simulink library "Mylibrary"  (Simulink 8.3)
settings: Solver=ode45  StartTime=0.0  StopTime=10.0  RelTol=1e-3
undefined symbols (not defined in the file or in its folder): Delay, epsilon, L, Mode, R, T_Trigger, tau_bar, Ts, Ts1, vd, Vehicle_Index, vp, x0, y0
undefined symbols (not defined in the file): d1, m1, psi20, Vx, Vy, x20, y20
libraries: Mylibrary x3
(part 3 of 3)

== matlab function CPF Lapier Miguel Hung  ==
  settings: updateMethod=DISCRETE  sampleTime=0.2
  data: t input double; Re_Data1 input double; Re_Data2 input double; Com_Sig input double; tau_bar parameter double; DataToTran output double; p input double size=2; r input double; yaw input double size=1; u input double size=1; gamma_c output double size=1; vcxy_hat output double; yaw_ref output double; r_ref output double; precise output double; u_ref output double; pd output double; L parameter double; R parameter double; d parameter double; m parameter double; vp parameter double; gamma_dot output double
function [DataToTran,gamma_c,vcxy_hat,yaw_ref,r_ref,precise,u_ref,pd,gamma_dot] = fcn(t,Re_Data1,Re_Data2,Com_Sig,tau_bar,p,r,yaw,u,L, R, d, m, vp)
%% declare variables
    persistent  gamma gamma_c_M 
    persistent vcx vcy
    if isempty (gamma)
         gamma=0; gamma_c_M=0;                                 % we can start any value of gamma here
         vcx=0;vcy=0;
    end
%% In first 2 seconds, do nothing, just wait for estimation of GPS, sensors    
    if t<2
        DataToTran=[0;0];
        gamma_c=0;
        vcxy_hat=[0;0];
        yaw_ref=0;
        r_ref=0;
        precise=0;
        u_ref=0;    
        pd=[0;0];
        gamma_dot=0;
    else
%% After two senconds, do the job    
%-------------------
    Ts=0.2; 
% Update the path and coordination state gamma_c
    [gamma_c,vd_bar,path_point] = path(gamma,L, R, d, m, vp);
    pd=[path_point(1);path_point(2)]; 
    theta_c=path_point(3)*180/pi;
    c_c=path_point(5);
    g_c=path_point(6);
    s_dot=path_point(7);
    s_ddot=path_point(8);
% Calculate correction speed from coordination law  
    v_comp=norm([vp*cosd(yaw)+vcx vp*sind(yaw)+vcy]);
    [vd_t,DataToTran] = Coordination(t,gamma_c,gamma_c_M,Re_Data1,Re_Data2,Com_Sig,tau_bar,vp,v_comp,vd_bar);
% Implement Path Following Controller
    vd=vd_bar+0*vd_t;
    [gamma_next,vcxy_hat,yaw_ref,r_ref,precise,u_ref,pd,gamma_dot] = PF(vd,p,r,yaw,u,theta_c,c_c,g_c,pd,s_dot,s_ddot,t);
% Update gamma_c_M
    gamma_c_M=gamma_c;
    gamma=gamma_next;
    vcx=vcxy_hat(1);
    vcy=vcxy_hat(2);
%---------------------
    end
end

function [gamma_next,vcxy_hat,yaw_ref,r_ref,precise,u_ref,pd,gamma_dot] = PF(vd,p,r,yaw,u,theta_c,c_c,g_c,pd,s_dot,s_ddot,t)

%% Declare and initialize global variales                                   These variables will be kept in memory during execuation
    Ts=0.2;         
    persistent vr_hat_old   vr_hat    % sampling time
    persistent p_hat_old    p_hat   Vcxy_hat_old Vcxy_hat 
    persistent gamma 
    if isempty(p_hat)
        vr_hat_old=0;            vr_hat=0; 
        p_hat=p;                 p_hat_old=p;    Vcxy_hat_old=[0;0];  Vcxy_hat=[0;0];
        gamma=0;  
    end    
%% Vehicle Prameters
    mass = 17.0;
    X_dot_u = -20;
    Y_dot_v = -30;                                                              %-1.3175;
    Y_v = -50;
    Y_vv = -0.01;                                                               %-101.2776;
    % masses
    m_u = mass - X_dot_u;
    m_v = mass - Y_dot_v;
    N_r = -4.14; %-0.1
    N_rr = -6.23; %-21
%% error between vehicle and rabbit
   R1=[cosd(theta_c)       sind(theta_c);     % From {I} to {F}
      -sind(theta_c)       cosd(theta_c)]; 
   e=p-pd;
   e_f=R1*e;
   s1=e_f(1);
   y1=e_f(2);      
%% Estimate vr
    d_v = -Y_v - Y_vv*abs(vr_hat);
    vr_hat_dot=-m_u*u*r/m_v-d_v*vr_hat/m_v;
    vr_hat=vr_hat_old+Ts*vr_hat_dot;
    vr_hat_old=vr_hat; 
%% Estimate current 
% Estimate current in Inertial frame
    R2=[cosd(yaw)        -sind(yaw);     % From {B} to {I}
        sind(yaw)         cosd(yaw)]; 
    p_t=p-p_hat;
    Vr=[u;0*vr_hat];
    Kp=10*[1 0;
           0 1];
    Kc=10*[1 0;
          0 1];
    p_hat_dot=R2*Vr+Vcxy_hat+Kp*p_t;
    p_hat=p_hat_old+Ts*p_hat_dot;
    p_hat_old=p_hat;
    Vcxy_hat_dot=Kc*p_t;
    Vcxy_hat=Vcxy_hat_old+Ts*Vcxy_hat_dot;
    Vcxy_hat_old=Vcxy_hat;
    vcxy_hat=Vcxy_hat;
% Transform the estimated current to Frenet frame
    Vc_hat_f=R1*Vcxy_hat;                      
    Vc_par=Vc_hat_f(1);
    Vc_per=Vc_hat_f(2);
%% Outerloop Controller
   s=8;
   if t<=20;
       m=0.05*t;
   else
       m=1;
   end
   a=y1/s+m*Vc_per/u;
%    a=y1/s;                                             % No current                          
   a= min(max(a, -1), 1);
   theta=-asind(a);
% Yaw reference
   yaw_ref=theta_c+theta;
%    yaw_ref=60;
% Yaw rate reference
    r_ref=-c_c*s_dot*180/pi;
%     r_ref=0;
% speed reference

%      R3=[cosd(yaw)         sind(yaw);     % From {B} to {I}
%          -sind(yaw)         cosd(yaw)]; 
     u_ref=vd;
%% Gamma Controller
   k1=1;
   gamma_dot=u*cosd(yaw-theta_c)+k1*s1+Vc_par;
%       gamma_dot=vd*cosd(yaw-theta_c)+k1*s1;
%    if gamma_dot<=0
%        gamma_dot=0;
%    end
   gamma_next=gamma+Ts*gamma_dot;
   gamma=gamma_next;
% Precicise 
    r_rad=r*pi/180;
    precise=-g_c*s_dot^2-c_c*s_ddot - N_r*r_rad - N_rr*r_rad*abs(r_rad);
%     precise=0;
end
%%-------------------------------------------------------------------------------------------------------------
%%-------------------------------------------------------------------------------------------------------------
function [vd_t,DataToTran,e_int] = Coordination(t,gamma_c,gamma_c_M,Re_Data1,Re_Data2,Com_Sig,tau_bar,vp,v_comp,vd_bar)

%% Declare variables
    persistent gamma_cn1 gamma_cn2 gamma_c0 tc1 tc2 tcn11 tcn12 tcn21 tcn22 tem_c tem_cn1 tem_cn2 reset_c reset_cn1 reset_cn2 e_int_t;   
    if isempty(gamma_cn1)
        gamma_cn1=0;gamma_cn2=0;
        gamma_c0=0;
        tcn11=t;tcn12=t;
        tcn21=t;tcn22=t;
        tc1=t;tc2=t;
        tem_c=t;
        tem_cn1=t;tem_cn2=t;
        reset_c=false;
        reset_cn1=false;
        reset_cn2=false;
        e_int_t=0;
    end
%% Reset estimator for gamma_c of first neighbor;
    if (Re_Data1(1)~=0)                                  % If recived new data, reset estimator that the current vehicle thinks about the neighbor vehicle
        tcn11=Re_Data1(1); 
        tem_cn1=Re_Data1(2);
        reset_cn1=true;
    end   
    if (t-tcn11>tau_bar)&&reset_cn1
        gamma_cn1=tem_cn1+vp*tau_bar;
%         gamma_cn1=tem_cn1+vd_bar*tau_bar;
        reset_cn1=false;
        tcn12=t;
    end
%% Reset estimator for gamma_c of second neighbor;
    if (Re_Data2(1)~=0)                                  % If recived new data, reset estimator that the current vehicle thinks about the neighbor vehicle
        tcn21=Re_Data2(1); 
        tem_cn2=Re_Data2(2);
        reset_cn2=true;
    end   
    if (t-tcn21>tau_bar)&&reset_cn2
        gamma_cn2=tem_cn2+vp*tau_bar;
%         gamma_cn2=tem_cn2+vd_bar*tau_bar;

        reset_cn2=false;
        tcn22=t;
    end
%% Reset estimator for gamma_c of current vehicle   % When it sends its coordinate state to neighbor, it needs to update its estimator too to synchoronize with the neighbor
    if (Com_Sig~=0)
        tc1=t;
        tem_c=gamma_c;
        reset_c=true;
    end
    if (t-tc1>tau_bar)&& reset_c
        gamma_c0=tem_c+vp*tau_bar;
%                 gamma_c0=tem_c+vd_bar*tau_bar;

        reset_c=false;
        tc2=t;
    end
%% Run estimators of gamma
       gamma_c_hat=gamma_c0+vp*(t-tc2);
       gamma_c_n1_hat=gamma_cn1+vp*(t-tcn12);
       gamma_c_n2_hat=gamma_cn2+vp*(t-tcn22);
%      gamma_c_hat=gamma_c0+vd_bar*(t-tc2);
%      gamma_c_n1_hat=gamma_cn1+vd_bar*(t-tcn12);
%      gamma_c_n2_hat=gamma_cn2+vd_bar*(t-tcn22);
%% Accumulate error for integration term
    Ts=0.2;
    if (Re_Data1(2)~=0)                                                    % accumulate error when recieve new data from neigbor
       e=gamma_c_M-Re_Data1(2);
       e_int_t=e_int_t+.5*Ts*e;
    end
    if (Re_Data2(2)~=0) 
       e=gamma_c_M-Re_Data2(2);
       e_int_t=e_int_t+.5*Ts*e;
    end
%% Compute correction term 
    kg=.1;
    ki=.00;
    e1=(gamma_c_M-0.5*(gamma_c_n1_hat+gamma_c_n2_hat));
%     e1=(gamma_c_M-0.5*(Re_Data1(2)+Re_Data2(2)));
    vd_t=-kg*e1-ki*e_int_t;
    vd_t_max=vp;
    vd_t_min=-vp;
    if  vd_t<vd_t_min;
        vd_t=vd_t_min;
    elseif vd_t>=vd_t_max
        vd_t=vd_t_max;
    end
    e_int=e_int_t;
%% Prepare Data for transmition block
    gamma_e=gamma_c-gamma_c_hat;
    DataToTran=[gamma_c;gamma_e];
end
%%-------------------------------------------------------------------------------------------------------------
%%-------------------------------------------------------------------------------------------------------------
function [gamma_c,vd_bar,path_point] = path(gamma,L, R, d, m, vp) 
%% Path parameters
Ts=0.2;
s1=L-m;
s2=s1+pi*(R-d);
s3=s2+L;
s4=s3+pi*(R+d);
s5=s4+m;
ratio1=(R-d)/R;
ratio2=(R+d)/R;
% ratio1=1;
% ratio2=1;
if gamma<s5;
    cycle=0;
else
    cycle=1;
end
s=gamma-s5*cycle;
%% Declaration variable to calculate s_dot, s_ddot
persistent c_c_old gamma_old s_dot_old
if isempty(c_c_old)
    c_c_old=0;
    gamma_old=0;
    s_dot_old=0;
end
%% Update path information depending upon on gamma (or s)
if s<s1                                    % first segment of straight line;
    vd_bar=vp;
    xd=0+d;
    yd=s+R+m;
    theta_c=pi/2;
    gamma_c=s+s5*cycle;                    % the segment is parallel with x
    c_c=0;
elseif (s>=s1) && (s<=s2)                  % second segment, a circumference 
    vd_bar=ratio1*vp;
    theta_c=pi/2-(s-s1)/((R-d));
    xd=d+(R-d)*(1-sin(theta_c));
    yd=L+R+(R-d)*cos(theta_c);   
    gamma_c=s1+(s-s1)*R/(R-d)+s5*cycle; 
    c_c=1/(R-d);
elseif (s>s2) && (s<=s3)                   % third segment, a straight line 
    vd_bar=vp;
    yd=s3-s+R;  
    theta_c=-pi/2;
    xd=d+2*(R-d);
    gamma_c=s+d*pi+s5*cycle;
    c_c=0;
elseif (s>s3) && (s<=s4)   
    vd_bar=ratio2*vp;
    theta_c=-pi/2+(s-s3)/(R+d);
    xd=d+2*(R-d)+(R+d)*(1+sin(theta_c));
    yd=R-(R+d)*cos(theta_c);
    gamma_c=s3+d*pi+(s-s3)*R/(R+d)+s5*cycle;   
    c_c=-1/(R+d);
else
    vd_bar=vp;
    yd=(s-s4)+R;
    xd=d+4*R;
    theta_c=pi;
    gamma_c=s+s5*cycle;
    c_c=0;
end
%% Caculate s_dot,sddot,g_c

c_c_dot=c_c-c_c_old;
s_dot=(gamma-gamma_old)/Ts;
s_ddot=(s_dot-s_dot_old)/Ts;
                                                        % g_c=c_c_dot/s_dot;
if s_dot==0
    g_c=0;
else
    g_c=c_c_dot/s_dot; 
end   
%%      
c_c_old=c_c;
gamma_old=gamma;
s_dot_old=s_dot;
path_point=[cycle*4*R+xd,yd,theta_c,gamma,c_c,g_c,s_dot,s_ddot];
end

== matlab function CPF Lapier Miguel Hung Current ==
  settings: updateMethod=DISCRETE  sampleTime=0.2
  data: t input double; Re_Data1 input double; Re_Data2 input double; Com_Sig input double; tau_bar parameter double; DataToTran output double; p input double size=2; r input double; yaw input double size=1; u input double size=1; gamma_c output double size=1; vcxy_hat output double; yaw_ref output double; r_ref output double; precise output double; u_ref output double; pd output double; L parameter double; R parameter double; d parameter double; m parameter double; vp parameter double; gamma_dot output double
function [DataToTran,gamma_c,vcxy_hat,yaw_ref,r_ref,precise,u_ref,pd,gamma_dot] = fcn(t,Re_Data1,Re_Data2,Com_Sig,tau_bar,p,r,yaw,u,L, R, d, m, vp)
%% declare variables
    persistent  gamma gamma_c_M 
    persistent vcx vcy
    if isempty (gamma)
         gamma=0; gamma_c_M=0;                                 % we can start any value of gamma here
         vcx=0;vcy=0;
    end
%% In first 2 seconds, do nothing, just wait for estimation of GPS, sensors    
    if t<2
        DataToTran=[0;0];
        gamma_c=0;
        vcxy_hat=[0;0];
        yaw_ref=0;
        r_ref=0;
        precise=0;
        u_ref=0;    
        pd=[0;0];
        gamma_dot=0;
    else
%% After two senconds, do the job    
%-------------------
    Ts=0.2; 
% Update the path and coordination state gamma_c
    [gamma_c,vd_bar,path_point] = path(gamma,L, R, d, m, vp);
    pd=[path_point(1);path_point(2)]; 
    theta_c=path_point(3)*180/pi;
    c_c=path_point(5);
    g_c=path_point(6);
    s_dot=path_point(7);
    s_ddot=path_point(8);
% Calculate correction speed from coordination law  
    v_comp=norm([vp*cosd(yaw)+vcx vp*sind(yaw)+vcy]);
    [vd_t,DataToTran] = Coordination(t,gamma_c,gamma_c_M,Re_Data1,Re_Data2,Com_Sig,tau_bar,vp,v_comp,vd_bar);
% Implement Path Following Controller
    vd=vd_bar+0*vd_t;
    [gamma_next,vcxy_hat,yaw_ref,r_ref,precise,u_ref,pd,gamma_dot] = PF(vd,p,r,yaw,u,theta_c,c_c,g_c,pd,s_dot,s_ddot,t);
% Update gamma_c_M
    gamma_c_M=gamma_c;
    gamma=gamma_next;
    vcx=vcxy_hat(1);
    vcy=vcxy_hat(2);
%---------------------
    end
end

function [gamma_next,vcxy_hat,yaw_ref,r_ref,precise,u_ref,pd,gamma_dot] = PF(vd,p,r,yaw,u,theta_c,c_c,g_c,pd,s_dot,s_ddot,t)

%% Declare and initialize global variales                                   These variables will be kept in memory during execuation
    Ts=0.2;         
    persistent vr_hat_old   vr_hat    % sampling time
    persistent p_hat_old    p_hat   Vcxy_hat_old Vcxy_hat 
    persistent gamma 
    if isempty(p_hat)
        vr_hat_old=0;            vr_hat=0; 
        p_hat=p;                 p_hat_old=p;    Vcxy_hat_old=[0;0];  Vcxy_hat=[0;0];
        gamma=0;  
    end    
%% Vehicle Prameters
    mass = 17.0;
    X_dot_u = -20;
    Y_dot_v = -30;                                                              %-1.3175;
    Y_v = -50;
    Y_vv = -0.01;                                                               %-101.2776;
    % masses
    m_u = mass - X_dot_u;
    m_v = mass - Y_dot_v;
    N_r = -4.14; %-0.1
    N_rr = -6.23; %-21
%% error between vehicle and rabbit
   R1=[cosd(theta_c)       sind(theta_c);     % From {I} to {F}
      -sind(theta_c)       cosd(theta_c)]; 
   e=p-pd;
   e_f=R1*e;
   s1=e_f(1);
   y1=e_f(2);      
%% Estimate vr
    d_v = -Y_v - Y_vv*abs(vr_hat);
    vr_hat_dot=-m_u*u*r/m_v-d_v*vr_hat/m_v;
    vr_hat=vr_hat_old+Ts*vr_hat_dot;
    vr_hat_old=vr_hat; 
%% Estimate current 
% Estimate current in Inertial frame
    R2=[cosd(yaw)        -sind(yaw);     % From {B} to {I}
        sind(yaw)         cosd(yaw)]; 
    p_t=p-p_hat;
    Vr=[u;0*vr_hat];
    Kp=5*[1 0;
           0 1];
    Kc=5*[1 0;
          0 1];
    p_hat_dot=R2*Vr+Vcxy_hat+Kp*p_t;
    p_hat=p_hat_old+Ts*p_hat_dot;
    p_hat_old=p_hat;
    Vcxy_hat_dot=Kc*p_t;
    Vcxy_hat=Vcxy_hat_old+Ts*Vcxy_hat_dot;
    Vcxy_hat_old=Vcxy_hat;
    vcxy_hat=Vcxy_hat;

%% Outerloop Controller
   s=6;
   if t<=50;
       m=0.02*t;
   else
       m=1;
   end
   a=m*y1/s;
%    a=y1/s;                                             % No current                          
   a= min(max(a, -1), 1);
   % compute alpha
   phi_e=atan2d((u*sind(yaw)+Vcxy_hat(2)),(u*cosd(yaw)+Vcxy_hat(1)));
   alpha=phi_e-yaw; 
   beta_d=-asind(a);
   phi_e_ref=theta_c+beta_d;
% Yaw reference
   yaw_ref=phi_e_ref-alpha;
%    yaw_ref=60;
% Yaw rate reference
    r_ref=-c_c*s_dot*180/pi;
%     r_ref=0;
% speed reference

%      R3=[cosd(yaw)         sind(yaw);     % From {B} to {I}
%          -sind(yaw)         cosd(yaw)]; 
     u_ref=vd;
%% Gamma Controller
   k1=1;
   beta=phi_e-theta_c;
   gamma_dot=u_ref*cosd(beta)+k1*s1;
%       gamma_dot=vd*cosd(yaw-theta_c)+k1*s1;
%    if gamma_dot<=0
%        gamma_dot=0;
%    end
   gamma_next=gamma+Ts*gamma_dot;
   gamma=gamma_next;
% Precicise 
    r_rad=r*pi/180;
    precise=-g_c*s_dot^2-c_c*s_ddot - N_r*r_rad - N_rr*r_rad*abs(r_rad);
%     precise=0;
end
%%-------------------------------------------------------------------------------------------------------------
%%-------------------------------------------------------------------------------------------------------------
function [vd_t,DataToTran,e_int] = Coordination(t,gamma_c,gamma_c_M,Re_Data1,Re_Data2,Com_Sig,tau_bar,vp,v_comp,vd_bar)

%% Declare variables
    persistent gamma_cn1 gamma_cn2 gamma_c0 tc1 tc2 tcn11 tcn12 tcn21 tcn22 tem_c tem_cn1 tem_cn2 reset_c reset_cn1 reset_cn2 e_int_t;   
    if isempty(gamma_cn1)
        gamma_cn1=0;gamma_cn2=0;
        gamma_c0=0;
        tcn11=t;tcn12=t;
        tcn21=t;tcn22=t;
        tc1=t;tc2=t;
        tem_c=t;
        tem_cn1=t;tem_cn2=t;
        reset_c=false;
        reset_cn1=false;
        reset_cn2=false;
        e_int_t=0;
    end
%% Reset estimator for gamma_c of first neighbor;
    if (Re_Data1(1)~=0)                                  % If recived new data, reset estimator that the current vehicle thinks about the neighbor vehicle
        tcn11=Re_Data1(1); 
        tem_cn1=Re_Data1(2);
        reset_cn1=true;
    end   
    if (t-tcn11>tau_bar)&&reset_cn1
        gamma_cn1=tem_cn1+vp*tau_bar;
%         gamma_cn1=tem_cn1+vd_bar*tau_bar;
        reset_cn1=false;
        tcn12=t;
    end
%% Reset estimator for gamma_c of second neighbor;
    if (Re_Data2(1)~=0)                                  % If recived new data, reset estimator that the current vehicle thinks about the neighbor vehicle
        tcn21=Re_Data2(1); 
        tem_cn2=Re_Data2(2);
        reset_cn2=true;
    end   
    if (t-tcn21>tau_bar)&&reset_cn2
        gamma_cn2=tem_cn2+vp*tau_bar;
%         gamma_cn2=tem_cn2+vd_bar*tau_bar;

        reset_cn2=false;
        tcn22=t;
    end
%% Reset estimator for gamma_c of current vehicle   % When it sends its coordinate state to neighbor, it needs to update its estimator too to synchoronize with the neighbor
    if (Com_Sig~=0)
        tc1=t;
        tem_c=gamma_c;
        reset_c=true;
    end
    if (t-tc1>tau_bar)&& reset_c
        gamma_c0=tem_c+vp*tau_bar;
%                 gamma_c0=tem_c+vd_bar*tau_bar;

        reset_c=false;
        tc2=t;
    end
%% Run estimators of gamma
       gamma_c_hat=gamma_c0+vp*(t-tc2);
       gamma_c_n1_hat=gamma_cn1+vp*(t-tcn12);
       gamma_c_n2_hat=gamma_cn2+vp*(t-tcn22);
%      gamma_c_hat=gamma_c0+vd_bar*(t-tc2);
%      gamma_c_n1_hat=gamma_cn1+vd_bar*(t-tcn12);
%      gamma_c_n2_hat=gamma_cn2+vd_bar*(t-tcn22);
%% Accumulate error for integration term
    Ts=0.2;
    if (Re_Data1(2)~=0)                                                    % accumulate error when recieve new data from neigbor
       e=gamma_c_M-Re_Data1(2);
       e_int_t=e_int_t+.5*Ts*e;
    end
    if (Re_Data2(2)~=0) 
       e=gamma_c_M-Re_Data2(2);
       e_int_t=e_int_t+.5*Ts*e;
    end
%% Compute correction term 
    kg=.2;
    ki=.00;
    e1=(gamma_c_M-0.5*(gamma_c_n1_hat+gamma_c_n2_hat));
%     e1=(gamma_c_M-0.5*(Re_Data1(2)+Re_Data2(2)));
    vd_t=-kg*e1-ki*e_int_t;
    vd_t_max=vp;
    vd_t_min=-vp;
    if  vd_t<vd_t_min;
        vd_t=vd_t_min;
    elseif vd_t>=vd_t_max
        vd_t=vd_t_max;
    end
    e_int=e_int_t;
%% Prepare Data for transmition block
    gamma_e=gamma_c-gamma_c_hat;
    DataToTran=[gamma_c;gamma_e];
end
%%-------------------------------------------------------------------------------------------------------------
%%-------------------------------------------------------------------------------------------------------------
function [gamma_c,vd_bar,path_point] = path(gamma,L, R, d, m, vp) 
%% Path parameters
Ts=0.2;
s1=L-m;
s2=s1+pi*(R-d);
s3=s2+L;
s4=s3+pi*(R+d);
s5=s4+m;
ratio1=(R-d)/R;
ratio2=(R+d)/R;
% ratio1=1;
% ratio2=1;
if gamma<s5;
    cycle=0;
else
    cycle=1;
end
s=gamma-s5*cycle;
%% Declaration variable to calculate s_dot, s_ddot
persistent c_c_old gamma_old s_dot_old
if isempty(c_c_old)
    c_c_old=0;
    gamma_old=0;
    s_dot_old=0;
end
%% Update path information depending upon on gamma (or s)
if s<s1                                    % first segment of straight line;
    vd_bar=vp;
    xd=0+d;
    yd=s+R+m;
    theta_c=pi/2;
    gamma_c=s+s5*cycle;                    % the segment is parallel with x
    c_c=0;
elseif (s>=s1) && (s<=s2)                  % second segment, a circumference 
    vd_bar=ratio1*vp;
    theta_c=pi/2-(s-s1)/((R-d));
    xd=d+(R-d)*(1-sin(theta_c));
    yd=L+R+(R-d)*cos(theta_c);   
    gamma_c=s1+(s-s1)*R/(R-d)+s5*cycle; 
    c_c=1/(R-d);
elseif (s>s2) && (s<=s3)                   % third segment, a straight line 
    vd_bar=vp;
    yd=s3-s+R;  
    theta_c=-pi/2;
    xd=d+2*(R-d);
    gamma_c=s+d*pi+s5*cycle;
    c_c=0;
elseif (s>s3) && (s<=s4)   
    vd_bar=ratio2*vp;
    theta_c=-pi/2+(s-s3)/(R+d);
    xd=d+2*(R-d)+(R+d)*(1+sin(theta_c));
    yd=R-(R+d)*cos(theta_c);
    gamma_c=s3+d*pi+(s-s3)*R/(R+d)+s5*cycle;   
    c_c=-1/(R+d);
else
    vd_bar=vp;
    yd=(s-s4)+R;
    xd=d+4*R;
    theta_c=pi;
    gamma_c=s+s5*cycle;
    c_c=0;
end
%% Caculate s_dot,sddot,g_c

c_c_dot=c_c-c_c_old;
s_dot=(gamma-gamma_old)/Ts;
s_ddot=(s_dot-s_dot_old)/Ts;
                                                        % g_c=c_c_dot/s_dot;
if s_dot==0
    g_c=0;
else
    g_c=c_c_dot/s_dot; 
end   
%%      
c_c_old=c_c;
gamma_old=gamma;
s_dot_old=s_dot;
path_point=[cycle*4*R+xd,yd,theta_c,gamma,c_c,g_c,s_dot,s_ddot];
end

== matlab function Kinematic Model/Kinematic Model ==
  data: u input double; x_dot output double; yaw input double; y_dot output double
function [x_dot, y_dot] = fcn(u, yaw)
x_dot=u*cos(yaw);
y_dot=u*sin(yaw);

== matlab function Simplified CPF Controller Latest version  ==
  settings: updateMethod=DISCRETE  sampleTime=0.2
  data: t input double size=1; Re_Data1 input double size=2; Re_Data2 input double size=2; u input double size=1; r input double size=1; yaw input double size=1; p input double size=2; L parameter double size=1; R parameter double size=1; d parameter double size=1; m parameter double size=1; u_d output double size=1; r_d output double size=1; Com_Mode output double size=1; Diff_Mode output double size=1; DatatoTran output double size=2; vd_t output double size=1; vp parameter double size=1; pd output double size=2; Mode parameter double; T_Trigger parameter double; epsilon parameter double; tau_bar parameter double
%% CPF is main function for Event/Time Trigger Coordinated Pathfollowing
function [u_d,r_d,Com_Mode,Diff_Mode,DatatoTran,vd_t,pd] = CPF(t,Re_Data1,Re_Data2,u,r,yaw,p,L, R, d,m,vp, Mode,T_Trigger,epsilon,tau_bar)
%% Declare variables
persistent  gamma gamma_c_M 
persistent  Com_Sig
if isempty (gamma)
         gamma=0; gamma_c_M=0;                                              % Noted that we can start any value of gamma here
         Com_Sig=0;   
end
if t<5                                                                      % Wait for update GPS... I am not sure, must be confirmed by experts            
    Com_Mode=0;Diff_Mode=0;
    DatatoTran=[0;0];  
    u_d=0;
    r_d=0;
    vd_t=0;
    pd=[0;0];
else
% Update the path and coordination state gamma_c
    [gamma_c,pd,pd_gamma,vd_bar,cur] = path(gamma,vp,L,R,d,m);
    
%% Calculate correction speed from coordination law
    Ts=0.2; 
    % Step 1: Run internal estimator to estimate neigbor's coordination state
     [gamma_c_hat,gamma_c_n1_hat,gamma_c_n2_hat] = Int_Est(t,gamma_c,Re_Data1,Re_Data2,vp,Com_Sig,tau_bar);   
    % Step 2: Call Coordination rule
      vd_t = Coordination(gamma_c,gamma_c_M,Re_Data1,Re_Data2,gamma_c_n1_hat,gamma_c_n2_hat,vp);

%% Transmit data (time and coordinated state (normalized) to neighbor)
  [DatatoTran,Com_Sig] = Trans(t,gamma_c,gamma_c_hat, Mode,T_Trigger,epsilon,tau_bar);
%% Implement Path Following Controller
%     vd_t=0;
  [gamma_next,u_d,r_d,Com_Mode,Diff_Mode] = PF(t,pd,pd_gamma,vd_bar,vd_t,u,r,yaw,p,Ts,cur);
    
%% Update
    gamma_c_M=gamma_c;
    gamma=gamma_next;
end
end
    %% PF function is for Path Flollowing Controller                                  
    function [gamma_next,u_d,r_d,Com_Mode,Diff_Mode] = PF(t,pd,pd_gamma,vd_bar,vd_t,u,r,yaw,p,Ts,cur)

    %% Declare and initialize global variales                                   These variables will be kept in memory during execuation
        persistent p_hat_old    p_hat   Vcxy_hat_old Vcxy_hat 
        persistent gamma_dot_old gamma_dot gamma_old
        persistent ud_t
        persistent eu_old Com_Mode_old
        persistent er_old Diff_Mode_old
        persistent vd_old vd_new
        if isempty(p_hat_old)
            p_hat=p;                p_hat_old=p;    Vcxy_hat_old=[0;0];  Vcxy_hat=[0;0];
            gamma_dot_old=0;        gamma_dot=0;    gamma_old=0;
            eu_old=0; Com_Mode_old=0;
            er_old=0; Diff_Mode_old=0;
            vd_old=0; vd_new=0;
            lock=0;
        end

    %% Calculate rotation matrix from body frame to inertial frame

        R=[cosd(yaw)   -sind(yaw);
           sind(yaw)    cosd(yaw)]; 

    %% Estimate current 
    % Estimate current in Inertial frame
        p_t=p-p_hat;
        Vr=[u;0];
        Kp=10*[1 0;
               0 1];
        Kc=10*[1 0;
              0 1];
        p_hat_dot=R*Vr+Vcxy_hat+Kp*p_t;
        p_hat=p_hat_old+Ts*p_hat_dot;
        p_hat_old=p_hat;
        Vcxy_hat_dot=Kc*p_t;
        Vcxy_hat=Vcxy_hat_old+Ts*Vcxy_hat_dot;
        Vcxy_hat_old=Vcxy_hat;
    % Transform the estimated current to Body frame
        Vc_hat=R'*Vcxy_hat;

    %% Outerloop Controller
        vd=vd_bar+vd_t;
        e_out=R'*(p-pd);
        delta=-0.2;
        Delta_inv= 1*[1    0;
                      0 -1/delta];     

        if t<30
            kx=0.01*t;
            ky=0.006*t;
            m=.0017*t;
        else
            kx=0.3;
            ky=0.2;
            m=0.05;
        end
         
          Kk=[kx+cur 0;
            0  ky+cur];
          ud_t=Delta_inv*(-Kk*tanh(e_out-[delta;0])-Vc_hat+R'*pd_gamma*vd);  
          n=1;
         
          ud=[n 0; 0 m+cur]*ud_t;
          u_d=ud(1);
          r_d=ud(2)*180/(pi); 
    %% Inner Loop Controller
        eu=u_d-u;
        er=r_d-r;
        % Speed controller
        Kp_u=30;
        KI_u=10;
        KD_u=0;
        Com_Mode=Kp_u*eu+(Ts*KI_u-Kp_u)*eu_old+Com_Mode_old;
        Com_Mode_old=Com_Mode;
        eu_old=eu;
        % Yaw rate controller
        Kp_r=10;
        KI_r=2;
        KD_r=0;
        Diff_Mode=Kp_r*er+(Ts*KI_r-Kp_r)*er_old+Diff_Mode_old;
        Diff_Mode_old=Diff_Mode;
        er_old=er;

    %% Gamma Controller
        kz=1;
        vd_dot=(vd_new-vd_old)/Ts;   
        vd_old=vd_new;
        gamma_ddot=-kz*(gamma_dot-vd_bar)+vd_dot+2*(e_out-[delta;0])'*R'*pd_gamma + 1*kz*vd_t; 
        gamma_dot=gamma_dot_old+Ts*gamma_ddot;
        gamma_next=gamma_old+Ts*gamma_dot;
        gamma_dot_old=gamma_dot;
        gamma_old=gamma_next;
    end                 
    %% Coordinaiton function is for Time/Event Trigger Cordination Law
    function vd_t = Coordination(gamma_c,gamma_c_M,Re_Data1,Re_Data2,gamma_c_n1_hat,gamma_c_n2_hat,vp)
       persistent e_int;
       if isempty (e_int)
           e_int=0;
       end
    %% Accumulate error for integration term
        Ts=0.2;
        if (Re_Data1(2)~=0)                                                    % accumulate error when recieve new data from neigbor
           e=gamma_c_M-Re_Data1(2);
           e_int=e_int+.5*Ts*e;
        end
        if (Re_Data2(2)~=0) 
           e=gamma_c_M-Re_Data2(2);
           e_int=e_int+.5*Ts*e;
        end
    %% Compute correction term 
        kg=.1;
        ki=.000;
        e1=(gamma_c-0.5*(gamma_c_n1_hat+gamma_c_n2_hat));
    %     e1=(gamma_c_M-0.5*(Re_Data1(2)+Re_Data2(2)));
        vd_t=-kg*e1-ki*e_int;
    %   Put saturation to avoid the vehicle return back.    
        vd_t_max=vp;
        vd_t_min=-vp;
        if  vd_t<vd_t_min;
            vd_t=vd_t_min;
        elseif vd_t>=vd_t_max
            vd_t=vd_t_max;
        end
    end
    %% Internal Estimator
    function [gamma_c_hat,gamma_c_n1_hat,gamma_c_n2_hat] = Int_Est(t,gamma_c,Re_Data1,Re_Data2,vp,Com_Sig,tau_bar)                                                       % No delay
    %% Declare variables
        persistent gamma_cn1 gamma_cn2 gamma_c0 tc2 tcn12 tcn22 tem_c tem_cn1 tem_cn2   
        if isempty(gamma_cn1)
            gamma_cn1=0;gamma_cn2=0;
            gamma_c0=0;
            tcn12=t;
            tcn22=t;
            tc2=t;
            tem_c=t;
            tem_cn1=t;tem_cn2=t;
        end
    %% Reset estimator for gamma_c of first neighbor;
        if (Re_Data1(1)~=0)                                  % If recived new data, reset estimator that the current vehicle thinks about the neighbor vehicle
            tem_cn1=Re_Data1(2);
            gamma_cn1=tem_cn1+vp*tau_bar;                    % Compensate tau_bar is the delay time for transmition 
            tcn12=t;
        end
    %% Reset estimator for gamma_c of second neighbor;
        if (Re_Data2(1)~=0)                                  % If recived new data, reset estimator that the current vehicle thinks about the neighbor vehicle
            tem_cn2=Re_Data2(2);
            gamma_cn2=tem_cn2+vp*tau_bar;
            tcn22=t;
        end
    %% Reset estimator for gamma_c of current vehicle        % When the vehicle sends its coordinate state to neighbors, it needs to update its estimator too to synchoronize with its neighbors
        if (Com_Sig~=0)
            tem_c=gamma_c;
            gamma_c0=tem_c;
            tc2=t;
        end
    %% Run estimators of gamma
        gamma_c_hat=gamma_c0+vp*(t-tc2);
        gamma_c_n1_hat=gamma_cn1+vp*(t-tcn12);
        gamma_c_n2_hat=gamma_cn2+vp*(t-tcn22); 
end
    %% Path function is path generator (Lawn mower)
    function [gamma_c,pd,pd_gamma,vd_bar,cur] = path(gamma,vp,L,R,d,m) 
    s1=L-m;
    s2=s1+pi*(R-d);
    s3=s2+L;
    s4=s3+pi*(R+d);
    s5=s4+m;
    ratio1=(R-d)/R;
    ratio2=(R+d)/R;
%     ratio1=1;
%     ratio2=1;

    if gamma<s5;
        cycle=0;
    else
        cycle=1;
    end
    s=gamma-s5*cycle;
    c1=1.2/(R-d);
    c2=1/(R+d);
    k=.5;
    cur=c1/(1+exp(-k*(s-s1)))-c1/(1+exp(-k*(s-s2)))+c2/(1+exp(-k*(s-s3)))-c2/(1+exp(-k*(s-s4)));
    if s<s1                                    % first segment of straight line;
        vd_bar=vp;
        xd=s+R+m;
        yd=0+d;
        pd_gamma=[1;0];      
        gamma_c=s+s5*cycle;                                  % the segment is parallel with x
    elseif (s>=s1) && (s<=s2)                  % second segment, a circumference 
        vd_bar=ratio1*vp;
        psi_T=(s-s1)/(R-d);
        xd=L+R+(R-d)*sin(psi_T);   
        yd=d+(R-d)*(1-cos(psi_T));
        pd_gamma=[cos(psi_T);sin(psi_T)];
        gamma_c=s1+(s-s1)*R/(R-d)+s5*cycle; 
    elseif (s>s2) && (s<=s3)                   % third segment, a straight line 
        vd_bar=vp;
        xd=s3-s+R;  
        yd=d+2*(R-d); 
        pd_gamma=[-1;0];
        gamma_c=s+d*pi+s5*cycle;
    elseif (s>s3) && (s<=s4)   
        vd_bar=ratio2*vp;
        xd=R-(R+d)*sin((s-s3)/(R+d));
        yd=d+2*(R-d)+(R+d)*(1-cos((s-s3)/(R+d)));
        pd_gamma=[-cos((s-s3)/(R+d));sin((s-s3)/(R+d))]; 
        gamma_c=s3+d*pi+(s-s3)*R/(R+d)+s5*cycle;  
    else
        vd_bar=vp;
        xd=(s-s4)+R;
        yd=d+4*R;
        pd_gamma=[1;0];
        gamma_c=s+s5*cycle;
    end
    if cycle ==0
        pd=[xd;cycle*4*R+yd];
    else 
        pd=[xd;cycle*4*R+yd];
    end
    %% Rotate the mission
    phi=pi/4;
    R=[cos(phi)   sin(phi);
       -sin(phi)  cos(phi)]; 
    pd=R*pd;
    pd_gamma=R*pd_gamma;
    end
    %% Trans is for trasmiting data to other vehicles
    function [DatatoTran,Com_Sig] = Trans(t,gamma_c,gamma_c_hat, Mode,T_Trigger,epsilon,tau_bar)
    %% Initialize temporary variables
        persistent t_sent;
        emptydata=[0;0];             
        gamma_e=gamma_c-gamma_c_hat;
        if isempty(t_sent);
            t_sent=-tau_bar;
            DatatoTran=emptydata;
            Com_Sig=0;
        else
            DatatoTran=emptydata;
            Com_Sig=1;
        end

        % Time trigger communication
        if Mode==1                                  
           if ~mod(t,T_Trigger)                           
                DatatoTran=[t;gamma_c];     
                t_sent=t;  % Include time in transmitted data
                Com_Sig=1;
           else
                DatatoTran=emptydata;
                Com_Sig=0;
           end           
        end
        % Event trigger communication
        T_wait=0.2;
        t_wait=t-t_sent;                            
        if Mode==2                                  
            if ((abs(gamma_e)>=epsilon)&&(t_wait>=T_wait));                 % Event trigger 
                t_sent=t;                                                   % Tag t to t_sent;     
                DatatoTran=[t;gamma_c];
                Com_Sig=1;
            else 
                DatatoTran=emptydata;
                Com_Sig=0;
            end
        end
    end

== matlab function CPF Controller Latest version for Test ==
  settings: updateMethod=DISCRETE  sampleTime=0.2
  data: t input double size=1; Data input double size=6; u input double size=1; r input double size=1; yaw input double size=1; p input double size=2; L parameter double size=1; R parameter double size=1; d parameter double size=1; m parameter double size=1; u_d output double size=1; r_d output double size=1; Com_Mode output double size=1; Diff_Mode output double size=1; DatatoTran output double size=3; vd_t output double size=1; vp parameter double size=1; pd output double size=2; Mode parameter double; T_Trigger parameter double; epsilon parameter double; tau_bar parameter double; V_Id parameter double
%% CPF is main function for Event/Time Trigger Coordinated Pathfollowing
function [u_d,r_d,Com_Mode,Diff_Mode,DatatoTran,vd_t,pd] = CPF(t,Data, u,r,yaw,p,L, R, d,m,vp, Mode,T_Trigger,epsilon,tau_bar,V_Id)
%% Declare variables
persistent  gamma gamma_c_M 
persistent  Com_Sig
if isempty (gamma)
         gamma=0; gamma_c_M=0;                                              % Noted that we can start any value of gamma here
         Com_Sig=0;   
end
if t<5                                                                      % Wait for update GPS... I am not sure, must be confirmed by experts            
    Com_Mode=0;Diff_Mode=0;
    DatatoTran=[V_Id;0;0];  
    u_d=0;
    r_d=0;
    vd_t=0;
    pd=[0;0];
else
%%   Check data in reciever 

    [Re_Data1,Re_Data2]=Reciever(Data,V_Id);
% Update the path and coordination state gamma_c
    [gamma_c,pd,pd_gamma,vd_bar,cur] = path(gamma,vp,L,R,d,m);
    
%% Calculate correction speed from coordination law
    Ts=0.2; 
    % Step 1: Run internal estimator to estimate neigbor's coordination state
     [gamma_c_hat,gamma_c_n1_hat,gamma_c_n2_hat] = Int_Est(t,gamma_c,Re_Data1,Re_Data2,vp,Com_Sig,tau_bar);   
    % Step 2: Call Coordination rule
      vd_t = Coordination(gamma_c,gamma_c_M,Re_Data1,Re_Data2,gamma_c_n1_hat,gamma_c_n2_hat,vp,V_Id);

%% Transmit data (time and coordinated state (normalized) to neighbor)
  [DatatoTran,Com_Sig] = Trans(t,gamma_c,gamma_c_hat, Mode,T_Trigger,epsilon,tau_bar,V_Id);
%% Implement Path Following Controller
%     vd_t=0;
  [gamma_next,u_d,r_d,Com_Mode,Diff_Mode] = PF(t,pd,pd_gamma,vd_bar,vd_t,u,r,yaw,p,Ts,cur);
    
%% Update
    gamma_c_M=gamma_c;
    gamma=gamma_next;
end
end
    %% PF function is for Path Flollowing Controller                                  
    function [gamma_next,u_d,r_d,Com_Mode,Diff_Mode] = PF(t,pd,pd_gamma,vd_bar,vd_t,u,r,yaw,p,Ts,cur)

    %% Declare and initialize global variales                                   These variables will be kept in memory during execuation
        persistent p_hat_old    p_hat   Vcxy_hat_old Vcxy_hat 
        persistent gamma_dot_old gamma_dot gamma_old
        persistent ud_t
        persistent eu_old Com_Mode_old
        persistent er_old Diff_Mode_old
        persistent vd_old vd_new
        if isempty(p_hat_old)
            p_hat=p;                p_hat_old=p;    Vcxy_hat_old=[0;0];  Vcxy_hat=[0;0];
            gamma_dot_old=0;        gamma_dot=0;    gamma_old=0;
            eu_old=0; Com_Mode_old=0;
            er_old=0; Diff_Mode_old=0;
            vd_old=0; vd_new=0;
            lock=0;
        end

    %% Calculate rotation matrix from body frame to inertial frame

        R=[cosd(yaw)   -sind(yaw);
           sind(yaw)    cosd(yaw)]; 

    %% Estimate current 
    % Estimate current in Inertial frame
        p_t=p-p_hat;
        Vr=[u;0];
        Kp=10*[1 0;
               0 1];
        Kc=10*[1 0;
              0 1];
        p_hat_dot=R*Vr+Vcxy_hat+Kp*p_t;
        p_hat=p_hat_old+Ts*p_hat_dot;
        p_hat_old=p_hat;
        Vcxy_hat_dot=Kc*p_t;
        Vcxy_hat=Vcxy_hat_old+Ts*Vcxy_hat_dot;
        Vcxy_hat_old=Vcxy_hat;
    % Transform the estimated current to Body frame
        Vc_hat=R'*Vcxy_hat;

    %% Outerloop Controller
        vd=vd_bar+vd_t;
        e_out=R'*(p-pd);
        delta=-0.2;
        Delta_inv= 1*[1    0;
                      0 -1/delta];     

        if t<30
            kx=0.01*t;
            ky=0.006*t;
            m=.0017*t;
        else
            kx=0.3;
            ky=0.2;
            m=0.05;
        end
         
          Kk=[kx+cur 0;
            0  ky+cur];
          ud_t=Delta_inv*(-Kk*tanh(e_out-[delta;0])-Vc_hat+R'*pd_gamma*vd);  
          n=1;
         
          ud=[n 0; 0 m+cur]*ud_t;
          u_d=ud(1);
          r_d=ud(2)*180/(pi); 
    %% Inner Loop Controller
        eu=u_d-u;
        er=r_d-r;
        % Speed controller
        Kp_u=30;
        KI_u=10;
        KD_u=0;
        Com_Mode=Kp_u*eu+(Ts*KI_u-Kp_u)*eu_old+Com_Mode_old;
        Com_Mode_old=Com_Mode;
        eu_old=eu;
        % Yaw rate controller
        Kp_r=10;
        KI_r=2;
        KD_r=0;
        Diff_Mode=Kp_r*er+(Ts*KI_r-Kp_r)*er_old+Diff_Mode_old;
        Diff_Mode_old=Diff_Mode;
        er_old=er;

    %% Gamma Controller
        kz=1;
        vd_dot=(vd_new-vd_old)/Ts;   
        vd_old=vd_new;
        gamma_ddot=-kz*(gamma_dot-vd_bar)+vd_dot+2*(e_out-[delta;0])'*R'*pd_gamma + 1*kz*vd_t; 
        gamma_dot=gamma_dot_old+Ts*gamma_ddot;
        gamma_next=gamma_old+Ts*gamma_dot;
        gamma_dot_old=gamma_dot;
        gamma_old=gamma_next;
    end                 
    %% Coordinaiton function is for Time/Event Trigger Cordination Law
    function vd_t = Coordination(gamma_c,gamma_c_M,Re_Data1,Re_Data2,gamma_c_n1_hat,gamma_c_n2_hat,vp,V_Id)
       persistent e_int;
       if isempty (e_int)
           e_int=0;
       end
    %% Accumulate error for integration term
        Ts=0.2;
        if (Re_Data1(2)~=0)                                                    % accumulate error when recieve new data from neigbor
           e=gamma_c_M-Re_Data1(2);
           e_int=e_int+.5*Ts*e;
        end
        if (Re_Data2(2)~=0) 
           e=gamma_c_M-Re_Data2(2);
           e_int=e_int+.5*Ts*e;
        end
    %% Compute correction term 
        kg=.1;
        ki=.000;
        
        if V_Id==1      
            e1=(gamma_c-0.5*(gamma_c_n1_hat+gamma_c_n2_hat));
        else
            e1=gamma_c-gamma_c_n1_hat;
        end
    %     e1=(gamma_c_M-0.5*(Re_Data1(2)+Re_Data2(2)));
        vd_t=-kg*e1-ki*e_int;
    %   Put saturation to avoid the vehicle return back.    
        vd_t_max=vp;
        vd_t_min=-vp;
        if  vd_t<vd_t_min;
            vd_t=vd_t_min;
        elseif vd_t>=vd_t_max
            vd_t=vd_t_max;
        end
    end
    %% Internal Estimator
    function [gamma_c_hat,gamma_c_n1_hat,gamma_c_n2_hat] = Int_Est(t,gamma_c,Re_Data1,Re_Data2,vp,Com_Sig,tau_bar)                                                       % No delay
    %% Declare variables
        persistent gamma_cn1 gamma_cn2 gamma_c0 tc2 tcn12 tcn22 tem_c tem_cn1 tem_cn2   
        if isempty(gamma_cn1)
            gamma_cn1=0;gamma_cn2=0;
            gamma_c0=0;
            tcn12=t;
            tcn22=t;
            tc2=t;
            tem_c=t;
            tem_cn1=t;tem_cn2=t;
        end
    %% Reset estimator for gamma_c of first neighbor;
        if (Re_Data1(1)~=0)                                  % If recived new data, reset estimator that the current vehicle thinks about the neighbor vehicle
            tem_cn1=Re_Data1(2);
            gamma_cn1=tem_cn1+vp*tau_bar;                    % Compensate tau_bar is the delay time for transmition 
            tcn12=t;
        end
    %% Reset estimator for gamma_c of second neighbor;
        if (Re_Data2(1)~=0)                                  % If recived new data, reset estimator that the current vehicle thinks about the neighbor vehicle
            tem_cn2=Re_Data2(2);
            gamma_cn2=tem_cn2+vp*tau_bar;
            tcn22=t;
        end
    %% Reset estimator for gamma_c of current vehicle        % When the vehicle sends its coordinate state to neighbors, it needs to update its estimator too to synchoronize with its neighbors
        if (Com_Sig~=0)
            tem_c=gamma_c;
            gamma_c0=tem_c;
            tc2=t;
        end
    %% Run estimators of gamma
        gamma_c_hat=gamma_c0+vp*(t-tc2);
        gamma_c_n1_hat=gamma_cn1+vp*(t-tcn12);
        gamma_c_n2_hat=gamma_cn2+vp*(t-tcn22); 
end
    %% Path function is path generator (Lawn mower)
    function [gamma_c,pd,pd_gamma,vd_bar,cur] = path(gamma,vp,L,R,d,m) 
    s1=L-m;
    s2=s1+pi*(R-d);
    s3=s2+L;
    s4=s3+pi*(R+d);
    s5=s4+m;
    ratio1=(R-d)/R;
    ratio2=(R+d)/R;
%     ratio1=1;
%     ratio2=1;

    if gamma<s5;
        cycle=0;
    else
        cycle=1;
    end
    s=gamma-s5*cycle;
    c1=1.2/(R-d);
    c2=1/(R+d);
    k=.5;
    cur=c1/(1+exp(-k*(s-s1)))-c1/(1+exp(-k*(s-s2)))+c2/(1+exp(-k*(s-s3)))-c2/(1+exp(-k*(s-s4)));
    if s<s1                                    % first segment of straight line;
        vd_bar=vp;
        xd=s+R+m;
        yd=0+d;
        pd_gamma=[1;0];      
        gamma_c=s+s5*cycle;                                  % the segment is parallel with x
    elseif (s>=s1) && (s<=s2)                  % second segment, a circumference 
        vd_bar=ratio1*vp;
        psi_T=(s-s1)/(R-d);
        xd=L+R+(R-d)*sin(psi_T);   
        yd=d+(R-d)*(1-cos(psi_T));
        pd_gamma=[cos(psi_T);sin(psi_T)];
        gamma_c=s1+(s-s1)*R/(R-d)+s5*cycle; 
    elseif (s>s2) && (s<=s3)                   % third segment, a straight line 
        vd_bar=vp;
        xd=s3-s+R;  
        yd=d+2*(R-d); 
        pd_gamma=[-1;0];
        gamma_c=s+d*pi+s5*cycle;
    elseif (s>s3) && (s<=s4)   
        vd_bar=ratio2*vp;
        xd=R-(R+d)*sin((s-s3)/(R+d));
        yd=d+2*(R-d)+(R+d)*(1-cos((s-s3)/(R+d)));
        pd_gamma=[-cos((s-s3)/(R+d));sin((s-s3)/(R+d))]; 
        gamma_c=s3+d*pi+(s-s3)*R/(R+d)+s5*cycle;  
    else
        vd_bar=vp;
        xd=(s-s4)+R;
        yd=d+4*R;
        pd_gamma=[1;0];
        gamma_c=s+s5*cycle;
    end
    if cycle ==0
        pd=[xd;cycle*4*R+yd];
    else 
        pd=[xd;cycle*4*R+yd];
    end
    %% Rotate the mission
    phi=pi/4;
    R=[cos(phi)   sin(phi);
       -sin(phi)  cos(phi)]; 
    pd=R*pd;
    pd_gamma=R*pd_gamma;
    end
    %% Trans is for trasmiting data to other vehicles
    function [DatatoTran,Com_Sig] = Trans(t,gamma_c,gamma_c_hat, Mode,T_Trigger,epsilon,tau_bar,V_Id)
    %% Initialize temporary variables
        persistent t_sent;
        emptydata=[V_Id;0;0];             
        gamma_e=gamma_c-gamma_c_hat;
        if isempty(t_sent);
            t_sent=-tau_bar;
            DatatoTran=emptydata;
            Com_Sig=0;
        else
            DatatoTran=emptydata;
            Com_Sig=1;
        end

        % Time trigger communication
        if Mode==1                                  
           if ~mod(t,T_Trigger)                           
                DatatoTran=[V_Id;t;gamma_c];     
                t_sent=t;  % Include time in transmitted data
                Com_Sig=1;
           else
                DatatoTran=emptydata;
                Com_Sig=0;
           end           
        end
        % Event trigger communication
        T_wait=0.2;
        t_wait=t-t_sent;                            
        if Mode==2                                  
            if ((abs(gamma_e)>=epsilon)&&(t_wait>=T_wait));                 % Event trigger 
                t_sent=t;                                                   % Tag t to t_sent;     
                DatatoTran=[V_Id;t;gamma_c];
                Com_Sig=1;
            else 
                DatatoTran=emptydata;
                Com_Sig=0;
            end
        end
    end
    %% Recieve and classify communicaition information
    function [Re_Data1,Re_Data2] = Reciever(Data,V_Id)
        packet1=Data(1:3);
        packet2=Data(4:6);
        ID1=packet1(1);
        ID2=packet2(1);
        if V_Id==1                                                          %% Vehicle 1 has two neighbors 2 and 3
            if (ID1==2)
                Re_Data1=packet1(2:3);
            elseif(ID2==2)
                Re_Data1=packet2(2:3);
            else
                Re_Data1=[0;0];
            end
     
            if (ID1==3) 
                Re_Data2=packet1(2:3);            
            elseif(ID2==3) 
                Re_Data2=packet2(2:3);
            else
                Re_Data2=[0;0];
            end
    
        else                                                                %% Either vehicle 2 or 3 has only one neigbor 1
            if ID1==1
               Re_Data1=packet1(2:3);
               Re_Data2=[0;0;0];
            elseif ID2==1
                Re_Data1=packet2(2:3);
                Re_Data2=[0;0;0];
            else
                Re_Data1=[0;0;0];
                Re_Data2=[0;0;0];
            end
        end
    end

== matlab function  Real MEDUSA Vehicle (2013)/Medusa/Speed Controller /Embedded MATLAB Function1 ==
  data: Cm output double; Uref input double; Kpu parameter double; Kiu parameter double; qsiold input double; qsi output double; Vx input double; Vy input double; yaw input double; u output double; us input double; KSat parameter double
function [Cm, qsi, u] = controller(Uref, Kpu,Kiu, qsiold,Vx,Vy,yaw, us, KSat)
u=Vx*sind(yaw)+Vy*cosd(yaw);
err=u-Uref;
qsi=qsiold+err;

Cm=-Kpu*(err+us)-Kiu*qsi;
% Cm =+40*Uref-Kiu*qsi;
% if(t>10)
%     qsi=qsiold+err;
%     Cm =-Kpu*err-Kiu*qsi;
% end
if(abs(Cm) >= KSat)
   Cm = KSat*sign(Cm); 
   qsi = qsiold;
end
